simulink model "PI_1"  (R2018b)
settings: Solver=FixedStepDiscrete  StartTime=0.0  StopTime=10.0  RelTol=1e-3
settings Model: Creator=matlab  LastModifiedBy=matlab
settings DataIOCC: SaveOutput=off  SignalLogging=off  SaveTime=off
settings OptimizationCC: DefaultParameterBehavior=Inlined  EnhancedBackFolding=on  PassReuseOutputArgsAs=Individual arguments  OptimizeBlockOrder=speed  DifferentSizesBufferReuse=on  OptimizationCustomize=off
settings DebuggingCC: ParameterTunabilityLossMsg=error
settings SFSimCC: MATLABDynamicMemAlloc=off
settings RTWCC: SystemTargetFile=ert.tlc  TemplateMakefile=ert_default_tmf  PostCodeGenCommand=packNGo(buildInfo);  GenerateReport=on  IncludeHyperlinkInReport=on  LaunchReport=on  GenerateTraceInfo=on  GenerateTraceReport=on  GenerateTraceReportSl=on  GenerateTraceReportSf=on  GenerateTraceReportEml=on
settings CodeAppCC: ForceParamTrailComments=on  IgnoreCustomStorageClasses=off  OperatorAnnotations=on  SimulinkDataObjDesc=on  SFDataObjDesc=on  InsertBlockDesc=on
settings ERTTargetCC: TargetLangStandard=C99 (ISO)  GenerateSampleERTMain=on  InlinedParameterPlacement=NonHierarchical  ERTCustomFileTemplate=example_file_process.tlc

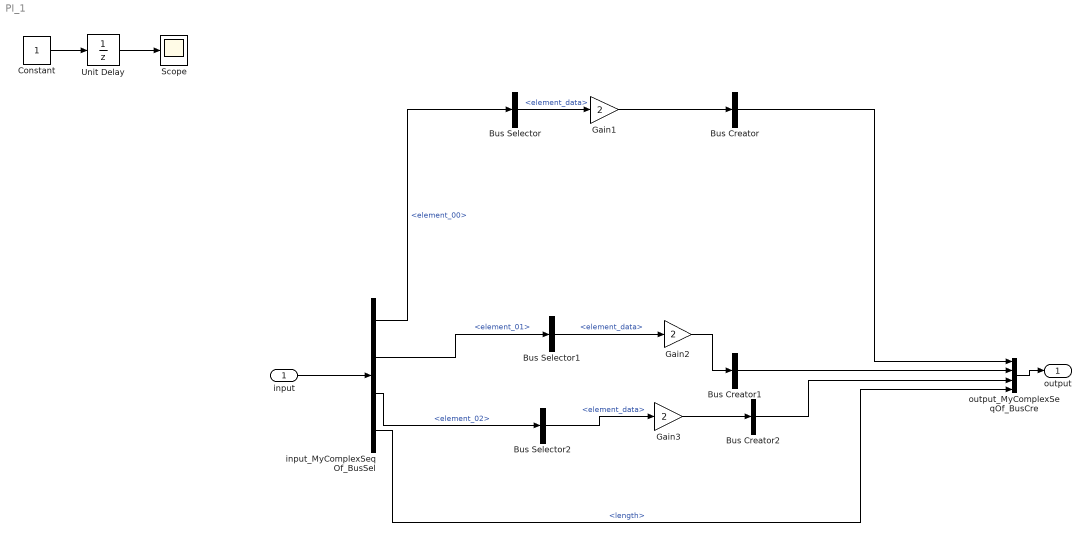
== system PI_1 ==
  input : Inport  OutDataTypeStr=Bus: MyComplexSeqOf  BusOutputAsStruct=on
  Bus Creator : BusCreator  Inputs=1  OutDataTypeStr=Bus: MySimpleSeqOf  NonVirtualBus=on
      settings: InheritFromInputs=off
  Bus Creator1 : BusCreator  Inputs=1  OutDataTypeStr=Bus: MySimpleSeqOf  NonVirtualBus=on
      settings: InheritFromInputs=off
  Bus Creator2 : BusCreator  Inputs=1  OutDataTypeStr=Bus: MySimpleSeqOf  NonVirtualBus=on
      settings: InheritFromInputs=off
  Bus Selector : BusSelector  OutputSignals=element_data
  Bus Selector1 : BusSelector  OutputSignals=element_data
  Bus Selector2 : BusSelector  OutputSignals=element_data
  Constant : Constant
  Gain1 : Gain  Gain=2  OutDataTypeStr=uint16
  Gain2 : Gain  Gain=2  OutDataTypeStr=uint16
  Gain3 : Gain  Gain=2  OutDataTypeStr=uint16
  Scope : Scope
  Unit Delay : UnitDelay  SampleTime=-1
  input_MyComplexSeqOf_BusSel : BusSelector  OutputSignals=element_00,element_01,element_02,length
  output_MyComplexSeqOf_BusCre : BusCreator  Inputs=4  OutDataTypeStr=Bus: MyComplexSeqOf  NonVirtualBus=on
      settings: InheritFromInputs=off
  output : Outport  OutDataTypeStr=Bus: MyComplexSeqOf  BusOutputAsStruct=on
  wires:
  input/1 -> input_MyComplexSeqOf_BusSel/1
  output_MyComplexSeqOf_BusCre/1 -> output/1
  input_MyComplexSeqOf_BusSel/4 -> output_MyComplexSeqOf_BusCre/4  "<length>"
  Unit Delay/1 -> Scope/1
  Constant/1 -> Unit Delay/1
  input_MyComplexSeqOf_BusSel/1 -> Bus Selector/1  "<element_00>"
  Gain1/1 -> Bus Creator/1
  Bus Creator/1 -> output_MyComplexSeqOf_BusCre/1
  Bus Creator1/1 -> output_MyComplexSeqOf_BusCre/2
  Bus Creator2/1 -> output_MyComplexSeqOf_BusCre/3
  Bus Selector/1 -> Gain1/1  "<element_data>"
  Bus Selector1/1 -> Gain2/1  "<element_data>"
  input_MyComplexSeqOf_BusSel/2 -> Bus Selector1/1  "<element_01>"
  Gain2/1 -> Bus Creator1/1
  Gain3/1 -> Bus Creator2/1
  Bus Selector2/1 -> Gain3/1  "<element_data>"
  input_MyComplexSeqOf_BusSel/3 -> Bus Selector2/1  "<element_02>"
